simulink model "LAB0_3"  (R2025b)
settings: Solver=ode3  StartTime=0.0  StopTime=20  FixedStep=0.001  RelTol=1e-3
values from neighbouring files (symbols this model uses):
  Kd = K(3)    [LAB0_compute_penalty (NOT USED).m]    (also in LAB0_design_controller.m = Kp * Td)
  Ki = K(2)    [LAB0_compute_penalty (NOT USED).m]    (also in LAB0_design_controller.m = Kp / Ti)
  Kp = K(1)    [LAB0_compute_penalty (NOT USED).m]    (also in LAB0_design_controller.m = Delta_K * cos(Delta_phi))
undefined symbols (not defined in the file or in its folder): degs2rpm, den_Hi, den_Hw, mot, National_Instruments, num_Hi, num_Hw, PCI, rpm2degs, sens, Tl
libraries: sldrtlib x3, simulink x3
settings Model: SimulationMode=external  ExtModeTrigDuration=100001  Creator=delpratogi  LastModifiedBy=Gioele
settings DataIOCC: ReturnWorkspaceOutputs=off
settings HardwareCC: ProdBitPerLong=64.0  ProdHWDeviceType=Intel->x86-64 (Linux 64)
settings RTWCC: SystemTargetFile=sldrt.tlc  TemplateMakefile=sldrt.tmf  RTWCompilerOptimization=on  Description=Simulink Desktop Real-Time
settings CodeAppCC: MaxIdLength=95.0
settings SimulinkDesktopRealTimeCC: ExtModeTransport=0.0  ExtModeStaticAllocSize=1000000.0  TargetLibSuffix=_sldrt.a  TargetPreCompLibLocation=C:\Program Files\MATLAB\R2025b\toolbox\sldrt\lib\win64  MultiwordLength=2048.0  DynamicStringBufferSize=256.0  ParMdlRefBuildCompliant=on  PreserveMATLABNamespacesInGeneratedCode=on  SubcomponentCodeInterfacePackaging=Reusable function

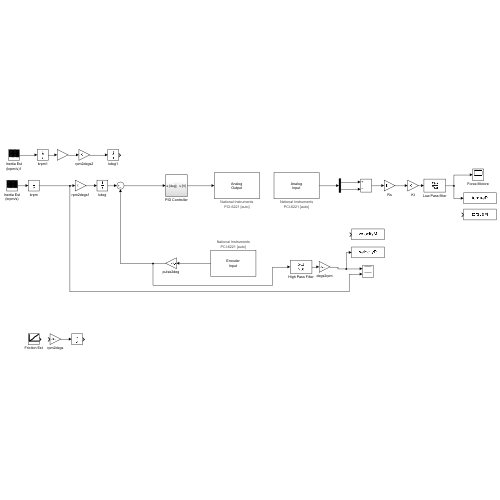
[thumbnail: Simulink's stored preview of the top-level diagram]
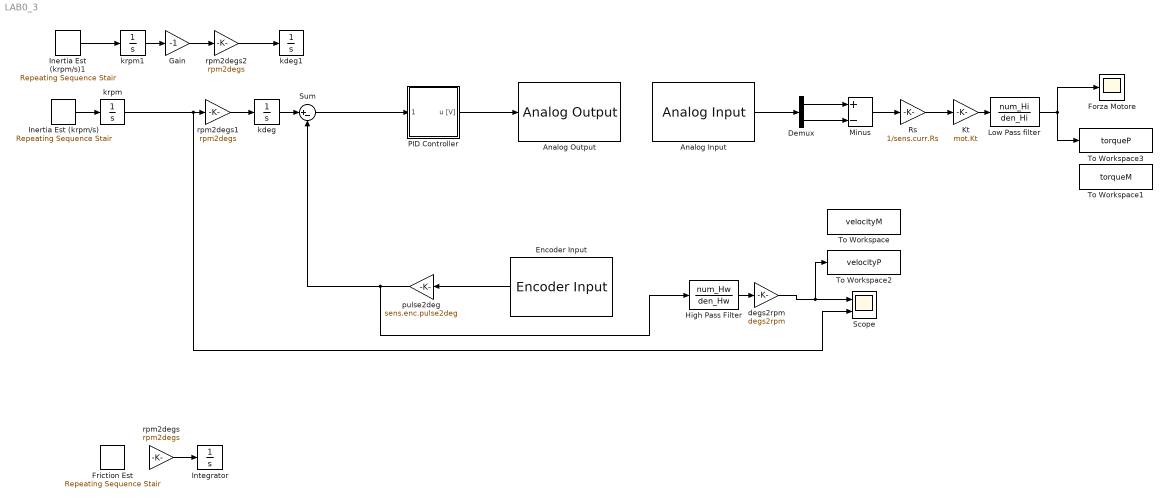
== system LAB0_3 ==
  Analog Input : sldrtlib/Analog Input  SampleTime=0.001  MaxMissedTicks=10  ShowMissedTicks=off  YieldWhenWaiting=off  DrvName=National_Instruments/PCI-6221  DrvAddress=4294967295  DrvOptions=[0 0 0 2 0]  Channels=[1,2]  RangeMode=1  VoltRange=1  DataType=1
      settings: AttributesFormatString=National Instruments\nPCI-6221 [auto]
  Analog Output : sldrtlib/Analog Output  SampleTime=0.001  MaxMissedTicks=10  ShowMissedTicks=off  YieldWhenWaiting=off  DrvName=National_Instruments/PCI-6221  DrvAddress=4294967295  DrvOptions=[0 0 0 2 0]  Channels=1  RangeMode=1  VoltRange=1  InitialValue=0  FinalValue=0
      settings: AttributesFormatString=National Instruments\nPCI-6221 [auto]
  Demux : Demux  Outputs=2
  Encoder Input : sldrtlib/Encoder Input  SampleTime=0.001  MaxMissedTicks=10  ShowMissedTicks=off  YieldWhenWaiting=off  DrvName=National_Instruments/PCI-6221  DrvAddress=4294967295  DrvOptions=[0 0 0 2 0]  Channels=1  QuadMode=3  IndexPulse=1  InputFilter=Inf  DataType=1
      settings: AttributesFormatString=National Instruments\nPCI-6221 [auto]
  Forza Motore : Scope
      settings: ActiveDisplayYMinimum=-0.00301  ActiveDisplayYMaximum=0.00033
  Friction Est : simulink/Sources/Repeating Sequence Stair  OutValues=stair_rpm  tsamp=5  OutMin=[]  OutMax=[]  OutDataTypeStr=double  OutputDataTypeScalingMode=double  OutDataType=fixdt(0,8)  ConRadixGroup=Best Precision: Vector-wise  OutScaling=2^-12
  Gain : Gain  Gain=-1
  High Pass Filter : TransferFcn  Numerator=num_Hw  Denominator=den_Hw
  Inertia Est (krpm/s) : simulink/Sources/Repeating Sequence Stair  OutValues="[450 -450 450 -450 450 -450  450 -450 450 -450 450 -450 450 -450 450 -450  450 -450 450 -450].'"  tsamp=1  OutMin=[]  OutMax=[]  OutDataTypeStr=double  OutputDataTypeScalingMode=double  OutDataType=fixdt(0,8)  ConRadixGroup=Best Precision: Vector-wise  OutScaling=2^-12
  Inertia Est (krpm/s)1 : simulink/Sources/Repeating Sequence Stair  OutValues="[450 -450 450 -450 450 -450  450 -450 450 -450 450 -450 450 -450 450 -450  450 -450 450 -450].'"  tsamp=1  OutMin=[]  OutMax=[]  OutDataTypeStr=double  OutputDataTypeScalingMode=double  OutDataType=fixdt(0,8)  ConRadixGroup=Best Precision: Vector-wise  OutScaling=2^-12
  Integrator : Integrator
  Kt : Gain  Gain=mot.Kt
  Low Pass filter : TransferFcn  Numerator=num_Hi  Denominator=den_Hi
  Minus : Sum  Inputs=+-
  PID Controller : Subsystem
  Rs : Gain  Gain=1/sens.curr.Rs
  Scope : Scope  NumInputPorts=2
      settings: ActiveDisplayYMinimum=-509.95865  ActiveDisplayYMaximum=509.46114
  Sum : Sum  Inputs=|+-
  To Workspace : ToWorkspace  VariableName=velocityM  SaveFormat=Structure With Time  SampleTime=-1
  To Workspace1 : ToWorkspace  VariableName=torqueM  SaveFormat=Structure With Time  SampleTime=-1
  To Workspace2 : ToWorkspace  VariableName=velocityP  SaveFormat=Timeseries  SampleTime=-1
  To Workspace3 : ToWorkspace  VariableName=torqueP  SaveFormat=Timeseries  SampleTime=-1
  degs2rpm : Gain  Gain=degs2rpm
  kdeg : Integrator
  kdeg1 : Integrator
  krpm : Integrator
  krpm1 : Integrator
  pulse2deg : Gain  Gain=sens.enc.pulse2deg
  rpm2degs : Gain  Gain=rpm2degs
  rpm2degs1 : Gain  Gain=rpm2degs
  rpm2degs2 : Gain  Gain=rpm2degs
  wires:
  PID Controller/1(u [V]) -> Analog Output/1
  Analog Input/1 -> Demux/1
  Demux/1 -> Minus/1
  Sum/1 -> PID Controller/1(e [deg])
  Encoder Input/1 -> pulse2deg/1
  Minus/1 -> Rs/1
  Demux/2 -> Minus/2
  Rs/1 -> Kt/1
  Low Pass filter/1 -> To Workspace3/1, Forza Motore/1
  Kt/1 -> Low Pass filter/1
  pulse2deg/1 -> High Pass Filter/1, Sum/2
  degs2rpm/1 -> To Workspace2/1, Scope/1
  High Pass Filter/1 -> degs2rpm/1
  rpm2degs/1 -> Integrator/1
  kdeg/1 -> Sum/1
  Inertia Est (krpm/s)/1 -> krpm/1
  rpm2degs1/1 -> kdeg/1
  krpm1/1 -> Gain/1
  rpm2degs2/1 -> kdeg1/1
  Gain/1 -> rpm2degs2/1
  Inertia Est (krpm/s)1/1 -> krpm1/1
  krpm/1 -> Scope/2, rpm2degs1/1

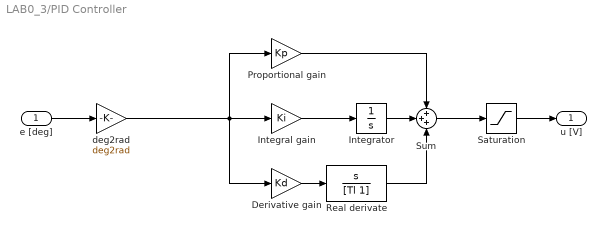
== system LAB0_3/PID Controller ==
  e [deg] : Inport
  Derivative gain : Gain  Gain=Kd
  "Integral gain " : Gain  Gain=Ki
  Integrator : Integrator
  Proportional gain : Gain  Gain=Kp
  Real derivate : TransferFcn  Numerator=[1 0]  Denominator=[Tl 1]
  Saturation : Saturate  UpperLimit=10  LowerLimit=-10
  Sum : Sum  Inputs=+++
  deg2rad : Gain  Gain=deg2rad
  u [V] : Outport
  wires:
  e [deg]/1 -> deg2rad/1
  Saturation/1 -> u [V]/1
  Sum/1 -> Saturation/1
  Integrator/1 -> Sum/2
  Derivative gain/1 -> Real derivate/1
  Proportional gain/1 -> Sum/1
  deg2rad/1 -> Proportional gain/1, Derivative gain/1, "Integral gain "/1
  "Integral gain "/1 -> Integrator/1
  Real derivate/1 -> Sum/3
